simulink model "PID_test"  (Simulink 7.9)
settings: Solver=ode45  StartTime=0.0  StopTime=10.0  RelTol=1e-3
settings Model: Creator=lenovo  LastModifiedBy=lenovo

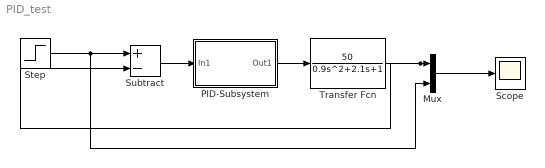
== system PID_test ==
  Mux : Mux  Inputs=2
  PID-Subsystem : Subsystem  mask{Gain_P=18, Gain_I=1, Gain_D=4}
      mask Display:
      | port_label('input',1,'Erro');
      | port_label('output',1,'Single');
      | image(imread('G:\Math Modeling\Matlab Development\Somematerial\PID_Log-1.png'));
  Scope : Scope
  Step : Step  SampleTime=0
  Subtract : Sum  Inputs=+-
  Transfer Fcn : TransferFcn  Numerator=[50]  Denominator=[0.9 2.1 1]
  wires:
  Mux/1 -> Scope/1
  PID-Subsystem/1(Out1) -> Transfer Fcn/1
  Step/1 -> Subtract/1, Mux/2
  Transfer Fcn/1 -> Mux/1, Subtract/2
  Subtract/1 -> PID-Subsystem/1(In1)

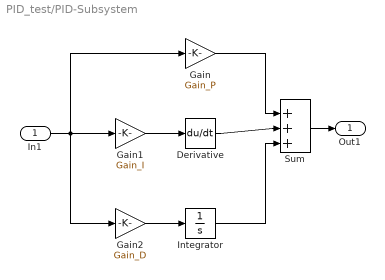
== system PID_test/PID-Subsystem ==
  In1 : Inport
  Derivative : Derivative
  Gain : Gain  Gain=Gain_P
  Gain1 : Gain  Gain=Gain_I
  Gain2 : Gain  Gain=Gain_D
  Integrator : Integrator
  Sum : Sum  Inputs=|+++
  Out1 : Outport
  wires:
  In1/1 -> Gain/1, Gain2/1, Gain1/1
  Gain1/1 -> Derivative/1
  Gain2/1 -> Integrator/1
  Gain/1 -> Sum/1
  Derivative/1 -> Sum/2
  Integrator/1 -> Sum/3
  Sum/1 -> Out1/1
